simulink model "Altitudecontrolnewscheme"  (R2016a)
settings: Solver=VariableStepAuto  StartTime=0.0  StopTime=10  FixedStep=Ts  RelTol=1e-3
model workspace (MAT data in the model file):
  AC_ATTITUDE_ACCEL_Y_CONTROLLER_MAX_RADSS = Simulink.Signal
  AC_ATTITUDE_ACCEL_Y_CONTROLLER_MAX_RADSS.DataType = 'double'
  AC_ATTITUDE_ACCEL_Y_CONTROLLER_MAX_RADSS.Dimensions = 1
  AC_ATTITUDE_ACCEL_Y_CONTROLLER_MAX_RADSS.DimensionsMode = 'auto'
  AC_ATTITUDE_ACCEL_Y_CONTROLLER_MAX_RADSS.Complexity = 'real'
  AC_ATTITUDE_ACCEL_Y_CONTROLLER_MAX_RADSS.SampleTime = -1
  AC_ATTITUDE_ACCEL_Y_CONTROLLER_MAX_RADSS.SamplingMode = 'Sample based'
  AC_ATTITUDE_ACCEL_Y_CONTROLLER_MAX_RADSS.InitialValue = '0.5'
  AC_ATTITUDE_CONTROL_MAX = Simulink.Signal
  AC_ATTITUDE_CONTROL_MAX.DataType = 'double'
  AC_ATTITUDE_CONTROL_MAX.Dimensions = 1
  AC_ATTITUDE_CONTROL_MAX.DimensionsMode = 'auto'
  AC_ATTITUDE_CONTROL_MAX.Complexity = 'real'
  AC_ATTITUDE_CONTROL_MAX.SampleTime = -1
  AC_ATTITUDE_CONTROL_MAX.SamplingMode = 'Sample based'
  AC_ATTITUDE_CONTROL_MAX.InitialValue = '0.5'
  AC_ATTITUDE_THRUST_ERROR_ANGLE = Simulink.Signal
  AC_ATTITUDE_THRUST_ERROR_ANGLE.DataType = 'double'
  AC_ATTITUDE_THRUST_ERROR_ANGLE.Dimensions = 1
  AC_ATTITUDE_THRUST_ERROR_ANGLE.DimensionsMode = 'auto'
  AC_ATTITUDE_THRUST_ERROR_ANGLE.Complexity = 'real'
  AC_ATTITUDE_THRUST_ERROR_ANGLE.SampleTime = -1
  AC_ATTITUDE_THRUST_ERROR_ANGLE.SamplingMode = 'Sample based'
  AC_ATTITUDE_THRUST_ERROR_ANGLE.InitialValue = '1000'
  ROLL_PITCH_INPUT_MAX = Simulink.Signal
  ROLL_PITCH_INPUT_MAX.DataType = 'double'
  ROLL_PITCH_INPUT_MAX.Dimensions = 1
  ROLL_PITCH_INPUT_MAX.DimensionsMode = 'auto'
  ROLL_PITCH_INPUT_MAX.Complexity = 'real'
  ROLL_PITCH_INPUT_MAX.SampleTime = -1
  ROLL_PITCH_INPUT_MAX.SamplingMode = 'Sample based'
  ROLL_PITCH_INPUT_MAX.InitialValue = '3000'
  Sig = Simulink.Signal
  Sig.DataType = 'auto'
  Sig.Dimensions = -1
  Sig.DimensionsMode = 'auto'
  Sig.Complexity = 'auto'
  Sig.SampleTime = -1
  Sig.SamplingMode = 'auto'
  Sig1 = Simulink.Signal
  Sig1.DataType = 'auto'
  Sig1.Dimensions = -1
  Sig1.DimensionsMode = 'auto'
  Sig1.Complexity = 'auto'
  Sig1.SampleTime = -1
  Sig1.SamplingMode = 'auto'
  acro_yaw_p = Simulink.Signal
  acro_yaw_p.DataType = 'double'
  acro_yaw_p.Dimensions = 1
  acro_yaw_p.DimensionsMode = 'auto'
  acro_yaw_p.Complexity = 'real'
  acro_yaw_p.SampleTime = -1
  acro_yaw_p.SamplingMode = 'Sample based'
  acro_yaw_p.InitialValue = '45'
  angle_max = Simulink.Signal
  angle_max.DataType = 'double'
  angle_max.Dimensions = 1
  angle_max.DimensionsMode = 'auto'
  angle_max.Complexity = 'real'
  angle_max.SampleTime = -1
  angle_max.SamplingMode = 'Sample based'
  angle_max.InitialValue = '3000'
  attitude_target_ang_vel = Simulink.Signal
  attitude_target_ang_vel.DataType = 'double'
  attitude_target_ang_vel.Dimensions = 3
  attitude_target_ang_vel.DimensionsMode = 'auto'
  attitude_target_ang_vel.Complexity = 'real'
  attitude_target_ang_vel.SampleTime = -1
  attitude_target_ang_vel.SamplingMode = 'Sample based'
  attitude_target_ang_vel.InitialValue = '[0 0 0]'
  attitude_target_euler_angle_x = Simulink.Signal
  attitude_target_euler_angle_x.DataType = 'double'
  attitude_target_euler_angle_x.Dimensions = 1
  attitude_target_euler_angle_x.DimensionsMode = 'auto'
  attitude_target_euler_angle_x.Complexity = 'real'
  attitude_target_euler_angle_x.SampleTime = -1
  attitude_target_euler_angle_x.SamplingMode = 'Sample based'
  attitude_target_euler_angle_x.InitialValue = '0'
  attitude_target_euler_angle_y = Simulink.Signal
  attitude_target_euler_angle_y.DataType = 'double'
  attitude_target_euler_angle_y.Dimensions = 1
  attitude_target_euler_angle_y.DimensionsMode = 'auto'
  attitude_target_euler_angle_y.Complexity = 'real'
  attitude_target_euler_angle_y.SampleTime = -1
  attitude_target_euler_angle_y.SamplingMode = 'Sample based'
  attitude_target_euler_angle_y.InitialValue = '0'
  attitude_target_euler_angle_z = Simulink.Signal
  attitude_target_euler_angle_z.DataType = 'double'
  attitude_target_euler_angle_z.Dimensions = 1
  attitude_target_euler_angle_z.DimensionsMode = 'auto'
  attitude_target_euler_angle_z.Complexity = 'real'
  attitude_target_euler_angle_z.SampleTime = -1
  attitude_target_euler_angle_z.SamplingMode = 'Sample based'
  attitude_target_euler_angle_z.InitialValue = '0'
  attitude_target_euler_rate = Simulink.Signal
  attitude_target_euler_rate.DataType = 'double'
  attitude_target_euler_rate.Dimensions = 3
  attitude_target_euler_rate.DimensionsMode = 'auto'
  attitude_target_euler_rate.Complexity = 'real'
  attitude_target_euler_rate.SampleTime = -1
  attitude_target_euler_rate.SamplingMode = 'Sample based'
  attitude_target_euler_rate.InitialValue = '[0 0 0]'
  attitude_target_quat = Simulink.Signal
  attitude_target_quat.DataType = 'double'
  attitude_target_quat.Dimensions = 4
  attitude_target_quat.DimensionsMode = 'auto'
  attitude_target_quat.Complexity = 'real'
  attitude_target_quat.SampleTime = -1
  attitude_target_quat.SamplingMode = 'Sample based'
  attitude_target_quat.InitialValue = '[1 0 0 0]'
  attitude_vehicle_quat = Simulink.Signal
  attitude_vehicle_quat.DataType = 'double'
  attitude_vehicle_quat.Dimensions = 4
  attitude_vehicle_quat.DimensionsMode = 'auto'
  attitude_vehicle_quat.Complexity = 'real'
  attitude_vehicle_quat.SampleTime = -1
  attitude_vehicle_quat.SamplingMode = 'Sample based'
  attitude_vehicle_quat.InitialValue = '[1 0 0 0]'
  dt = Simulink.Signal
  dt.DataType = 'double'
  dt.Dimensions = 1
  dt.DimensionsMode = 'auto'
  dt.Complexity = 'real'
  dt.SampleTime = -1
  dt.SamplingMode = 'Sample based'
  dt.InitialValue = '0.01'
  false = 0
  limit_roll_pitch = Simulink.Signal
  limit_roll_pitch.DataType = 'double'
  limit_roll_pitch.Dimensions = 1
  limit_roll_pitch.DimensionsMode = 'auto'
  limit_roll_pitch.Complexity = 'real'
  limit_roll_pitch.SampleTime = -1
  limit_roll_pitch.SamplingMode = 'Sample based'
  limit_roll_pitch.InitialValue = '0.0'
  limit_throttle_upper = Simulink.Signal
  limit_throttle_upper.DataType = 'logical'
  limit_throttle_upper.Dimensions = 1
  limit_throttle_upper.DimensionsMode = 'auto'
  limit_throttle_upper.Complexity = 'real'
  limit_throttle_upper.SampleTime = -1
  limit_throttle_upper.SamplingMode = 'Sample based'
  limit_throttle_upper.InitialValue = '0'
  limit_yaw = Simulink.Signal
  limit_yaw.DataType = 'double'
  limit_yaw.Dimensions = 1
  limit_yaw.DimensionsMode = 'auto'
  limit_yaw.Complexity = 'real'
  limit_yaw.SampleTime = -1
  limit_yaw.SamplingMode = 'Sample based'
  limit_yaw.InitialValue = '0'
  loop_rate = Simulink.Signal
  loop_rate.DataType = 'double'
  loop_rate.Dimensions = 1
  loop_rate.DimensionsMode = 'auto'
  loop_rate.Complexity = 'real'
  loop_rate.SampleTime = -1
  loop_rate.SamplingMode = 'Sample based'
  loop_rate.InitialValue = '100'
  pitch_attitude_kP = Simulink.Signal
  pitch_attitude_kP.DataType = 'double'
  pitch_attitude_kP.Dimensions = 1
  pitch_attitude_kP.DimensionsMode = 'auto'
  pitch_attitude_kP.Complexity = 'real'
  pitch_attitude_kP.SampleTime = -1
  pitch_attitude_kP.SamplingMode = 'Sample based'
  pitch_attitude_kP.InitialValue = '20'
  pitch_factor = Simulink.Signal
  pitch_factor.DataType = 'double'
  pitch_factor.Dimensions = 4
  pitch_factor.DimensionsMode = 'auto'
  pitch_factor.Complexity = 'real'
  pitch_factor.SampleTime = -1
  pitch_factor.SamplingMode = 'Sample based'
  pitch_factor.InitialValue = '[cos(deg2rad(15)) -cos(deg2rad(15)) cos(deg2rad(15)) -cos(deg2rad(15))]'
  pitch_rate_derivative = Simulink.Signal
  pitch_rate_derivative.DataType = 'double'
  pitch_rate_derivative.Dimensions = 1
  pitch_rate_derivative.DimensionsMode = 'auto'
  pitch_rate_derivative.Complexity = 'real'
  pitch_rate_derivative.SampleTime = -1
  pitch_rate_derivative.SamplingMode = 'Sample based'
  pitch_rate_derivative.InitialValue = '0'
  pitch_rate_error_rads = Simulink.Signal
  pitch_rate_error_rads.DataType = 'double'
  pitch_rate_error_rads.Dimensions = 1
  pitch_rate_error_rads.DimensionsMode = 'auto'
  pitch_rate_error_rads.Complexity = 'real'
  pitch_rate_error_rads.SampleTime = -1
  pitch_rate_error_rads.SamplingMode = 'Sample based'
  pitch_rate_error_rads.InitialValue = '0'
  pitch_rate_filt_hz = Simulink.Signal
  pitch_rate_filt_hz.DataType = 'double'
  pitch_rate_filt_hz.Dimensions = 1
  pitch_rate_filt_hz.DimensionsMode = 'auto'
  pitch_rate_filt_hz.Complexity = 'real'
  pitch_rate_filt_hz.SampleTime = -1
  pitch_rate_filt_hz.SamplingMode = 'Sample based'
  pitch_rate_filt_hz.InitialValue = '1/(2*pi)'
  pitch_rate_imax = Simulink.Signal
  pitch_rate_imax.DataType = 'double'
  pitch_rate_imax.Dimensions = 1
  pitch_rate_imax.DimensionsMode = 'auto'
  pitch_rate_imax.Complexity = 'real'
  pitch_rate_imax.SampleTime = -1
  pitch_rate_imax.SamplingMode = 'Sample based'
  pitch_rate_imax.InitialValue = '200'
  pitch_rate_integrator = Simulink.Signal
  pitch_rate_integrator.DataType = 'double'
  pitch_rate_integrator.Dimensions = 1
  pitch_rate_integrator.DimensionsMode = 'auto'
  pitch_rate_integrator.Complexity = 'real'
  pitch_rate_integrator.SampleTime = -1
  pitch_rate_integrator.SamplingMode = 'Sample based'
  pitch_rate_integrator.InitialValue = '0'
  pitch_rate_kD = Simulink.Signal
  pitch_rate_kD.DataType = 'double'
  pitch_rate_kD.Dimensions = 1
  pitch_rate_kD.DimensionsMode = 'auto'
  pitch_rate_kD.Complexity = 'real'
  pitch_rate_kD.SampleTime = -1
  pitch_rate_kD.SamplingMode = 'Sample based'
  pitch_rate_kD.InitialValue = '0.004'
  pitch_rate_kI = Simulink.Signal
  pitch_rate_kI.DataType = 'double'
  pitch_rate_kI.Dimensions = 1
  pitch_rate_kI.DimensionsMode = 'auto'
  pitch_rate_kI.Complexity = 'real'
  pitch_rate_kI.SampleTime = -1
  pitch_rate_kI.SamplingMode = 'Sample based'
  pitch_rate_kI.InitialValue = '0.1'
  pitch_rate_kP = Simulink.Signal
  pitch_rate_kP.DataType = 'double'
  pitch_rate_kP.Dimensions = 1
  pitch_rate_kP.DimensionsMode = 'auto'
  pitch_rate_kP.Complexity = 'real'
  pitch_rate_kP.SampleTime = -1
  pitch_rate_kP.SamplingMode = 'Sample based'
  pitch_rate_kP.InitialValue = '0.5'
  pitch_rate_last_input = Simulink.Signal
  pitch_rate_last_input.DataType = 'double'
  pitch_rate_last_input.Dimensions = 1
  pitch_rate_last_input.DimensionsMode = 'auto'
  pitch_rate_last_input.Complexity = 'real'
  pitch_rate_last_input.SampleTime = -1
  pitch_rate_last_input.SamplingMode = 'Sample based'
  pitch_rate_last_input.InitialValue = '0'
  pitch_rate_proportional = Simulink.Signal
  pitch_rate_proportional.DataType = 'double'
  pitch_rate_proportional.Dimensions = 1
  pitch_rate_proportional.DimensionsMode = 'auto'
  pitch_rate_proportional.Complexity = 'real'
  pitch_rate_proportional.SampleTime = -1
  pitch_rate_proportional.SamplingMode = 'Sample based'
  pitch_rate_proportional.InitialValue = '0'
  pwm_max = Simulink.Signal
  pwm_max.DataType = 'double'
  pwm_max.Dimensions = 1
  pwm_max.DimensionsMode = 'auto'
  pwm_max.Complexity = 'real'
  pwm_max.SampleTime = -1
  pwm_max.SamplingMode = 'Sample based'
  pwm_max.InitialValue = '2000'
  pwm_min = Simulink.Signal
  pwm_min.DataType = 'double'
  pwm_min.Dimensions = 1
  pwm_min.DimensionsMode = 'auto'
  pwm_min.Complexity = 'real'
  pwm_min.SampleTime = -1
  pwm_min.SamplingMode = 'Sample based'
  pwm_min.InitialValue = '1039'
  rate_bf_ff_enabled = Simulink.Signal
  rate_bf_ff_enabled.DataType = 'double'
  rate_bf_ff_enabled.Dimensions = 1
  rate_bf_ff_enabled.DimensionsMode = 'auto'
  rate_bf_ff_enabled.Complexity = 'real'
  rate_bf_ff_enabled.SampleTime = -1
  rate_bf_ff_enabled.SamplingMode = 'Sample based'
  rate_bf_ff_enabled.InitialValue = '0'
  rate_target_ang_vel = Simulink.Signal
  rate_target_ang_vel.DataType = 'double'
  rate_target_ang_vel.Dimensions = 3
  rate_target_ang_vel.DimensionsMode = 'auto'
  rate_target_ang_vel.Complexity = 'real'
  rate_target_ang_vel.SampleTime = -1
  rate_target_ang_vel.SamplingMode = 'Sample based'
  rate_target_ang_vel.InitialValue = '[0 0 0]'
  roll_attitude_kP = Simulink.Signal
  roll_attitude_kP.DataType = 'double'
  roll_attitude_kP.Dimensions = 1
  roll_attitude_kP.DimensionsMode = 'auto'
  roll_attitude_kP.Complexity = 'real'
  roll_attitude_kP.SampleTime = -1
  roll_attitude_kP.SamplingMode = 'Sample based'
  roll_attitude_kP.InitialValue = '20'
  roll_factor = Simulink.Signal
  roll_factor.DataType = 'double'
  roll_factor.Dimensions = 4
  roll_factor.DimensionsMode = 'auto'
  roll_factor.Complexity = 'real'
  roll_factor.SampleTime = -1
  roll_factor.SamplingMode = 'Sample based'
  roll_factor.InitialValue = '[-sin(deg2rad(15)) sin(deg2rad(15)) sin(deg2rad(15)) -sin(deg2rad(15))]'
  roll_rate_derivative = Simulink.Signal
  roll_rate_derivative.DataType = 'double'
  roll_rate_derivative.Dimensions = 1
  roll_rate_derivative.DimensionsMode = 'auto'
  roll_rate_derivative.Complexity = 'real'
  roll_rate_derivative.SampleTime = -1
  roll_rate_derivative.SamplingMode = 'Sample based'
  roll_rate_derivative.InitialValue = '0'
  roll_rate_error_rads = Simulink.Signal
  roll_rate_error_rads.DataType = 'double'
  roll_rate_error_rads.Dimensions = 1
  roll_rate_error_rads.DimensionsMode = 'auto'
  roll_rate_error_rads.Complexity = 'real'
  roll_rate_error_rads.SampleTime = -1
  roll_rate_error_rads.SamplingMode = 'Sample based'
  roll_rate_error_rads.InitialValue = '0'
  roll_rate_filt_hz = Simulink.Signal
  roll_rate_filt_hz.DataType = 'double'
  roll_rate_filt_hz.Dimensions = 1
  roll_rate_filt_hz.DimensionsMode = 'auto'
  roll_rate_filt_hz.Complexity = 'real'
  roll_rate_filt_hz.SampleTime = -1
  roll_rate_filt_hz.SamplingMode = 'Sample based'
  roll_rate_filt_hz.InitialValue = '1/(2*pi)'
  roll_rate_imax = Simulink.Signal
  roll_rate_imax.DataType = 'double'
  roll_rate_imax.Dimensions = 1
  roll_rate_imax.DimensionsMode = 'auto'
  roll_rate_imax.Complexity = 'real'
  roll_rate_imax.SampleTime = -1
  roll_rate_imax.SamplingMode = 'Sample based'
  roll_rate_imax.InitialValue = '200'
  roll_rate_integrator = Simulink.Signal
  roll_rate_integrator.DataType = 'double'
  roll_rate_integrator.Dimensions = 1
  roll_rate_integrator.DimensionsMode = 'auto'
  roll_rate_integrator.Complexity = 'real'
  roll_rate_integrator.SampleTime = -1
  roll_rate_integrator.SamplingMode = 'Sample based'
  roll_rate_integrator.InitialValue = '0'
  roll_rate_kD = Simulink.Signal
  roll_rate_kD.DataType = 'double'
  roll_rate_kD.Dimensions = 1
  roll_rate_kD.DimensionsMode = 'auto'
  roll_rate_kD.Complexity = 'real'
  roll_rate_kD.SampleTime = -1
  roll_rate_kD.SamplingMode = 'Sample based'
  roll_rate_kD.InitialValue = '0.004'
  roll_rate_kI = Simulink.Signal
  roll_rate_kI.DataType = 'double'
  roll_rate_kI.Dimensions = 1
  roll_rate_kI.DimensionsMode = 'auto'
  roll_rate_kI.Complexity = 'real'
  roll_rate_kI.SampleTime = -1
  roll_rate_kI.SamplingMode = 'Sample based'
  roll_rate_kI.InitialValue = '0.1'
  roll_rate_kP = Simulink.Signal
  roll_rate_kP.DataType = 'double'
  roll_rate_kP.Dimensions = 1
  roll_rate_kP.DimensionsMode = 'auto'
  roll_rate_kP.Complexity = 'real'
  roll_rate_kP.SampleTime = -1
  roll_rate_kP.SamplingMode = 'Sample based'
  roll_rate_kP.InitialValue = '1'
  roll_rate_last_input = Simulink.Signal
  roll_rate_last_input.DataType = 'double'
  roll_rate_last_input.Dimensions = 1
  roll_rate_last_input.DimensionsMode = 'auto'
  roll_rate_last_input.Complexity = 'real'
  roll_rate_last_input.SampleTime = -1
  roll_rate_last_input.SamplingMode = 'Sample based'
  roll_rate_last_input.InitialValue = '0'
  roll_rate_proportional = Simulink.Signal
  roll_rate_proportional.DataType = 'double'
  roll_rate_proportional.Dimensions = 1
  roll_rate_proportional.DimensionsMode = 'auto'
  roll_rate_proportional.Complexity = 'real'
  roll_rate_proportional.SampleTime = -1
  roll_rate_proportional.SamplingMode = 'Sample based'
  roll_rate_proportional.InitialValue = '0'
  spin_max = Simulink.Signal
  spin_max.DataType = 'double'
  spin_max.Dimensions = 1
  spin_max.DimensionsMode = 'auto'
  spin_max.Complexity = 'real'
  spin_max.SampleTime = -1
  spin_max.SamplingMode = 'Sample based'
  spin_max.InitialValue = '0.95'
  spin_min = Simulink.Signal
  spin_min.DataType = 'double'
  spin_min.Dimensions = 1
  spin_min.DimensionsMode = 'auto'
  spin_min.Complexity = 'real'
  spin_min.SampleTime = -1
  spin_min.SamplingMode = 'Sample based'
  spin_min.InitialValue = '0.15'
  throttle_avg_max = Simulink.Signal
  throttle_avg_max.DataType = 'double'
  throttle_avg_max.Dimensions = 1
  throttle_avg_max.DimensionsMode = 'auto'
  throttle_avg_max.Complexity = 'real'
  throttle_avg_max.SampleTime = -1
  throttle_avg_max.SamplingMode = 'Sample based'
  throttle_avg_max.InitialValue = '0'
  throttle_filter_cutoff_freq = Simulink.Signal
  throttle_filter_cutoff_freq.DataType = 'double'
  throttle_filter_cutoff_freq.Dimensions = 1
  throttle_filter_cutoff_freq.DimensionsMode = 'auto'
  throttle_filter_cutoff_freq.Complexity = 'real'
  throttle_filter_cutoff_freq.SampleTime = -1
  throttle_filter_cutoff_freq.SamplingMode = 'Sample based'
  throttle_filter_cutoff_freq.InitialValue = '0.5'
  throttle_filter_output = Simulink.Signal
  throttle_filter_output.DataType = 'double'
  throttle_filter_output.Dimensions = 1
  throttle_filter_output.DimensionsMode = 'auto'
  throttle_filter_output.Complexity = 'real'
  throttle_filter_output.SampleTime = -1
  throttle_filter_output.SamplingMode = 'Sample based'
  throttle_filter_output.InitialValue = '0'
  throttle_in = Simulink.Signal
  throttle_in.DataType = 'double'
  throttle_in.Dimensions = 1
  throttle_in.DimensionsMode = 'auto'
  throttle_in.Complexity = 'real'
  throttle_in.SampleTime = -1
  throttle_in.SamplingMode = 'Sample based'
  throttle_in.InitialValue = '0'
  throttle_rpy_mix = Simulink.Signal
  throttle_rpy_mix.DataType = 'double'
  throttle_rpy_mix.Dimensions = 1
  throttle_rpy_mix.DimensionsMode = 'auto'
  throttle_rpy_mix.Complexity = 'real'
  throttle_rpy_mix.SampleTime = -1
  throttle_rpy_mix.SamplingMode = 'Sample based'
  throttle_rpy_mix.InitialValue = '0'
  throttle_rpy_mix_desired = Simulink.Signal
  throttle_rpy_mix_desired.DataType = 'double'
  throttle_rpy_mix_desired.Dimensions = 1
  throttle_rpy_mix_desired.DimensionsMode = 'auto'
  throttle_rpy_mix_desired.Complexity = 'real'
  throttle_rpy_mix_desired.SampleTime = -1
  throttle_rpy_mix_desired.SamplingMode = 'Sample based'
  throttle_rpy_mix_desired.InitialValue = '0'
  throttle_thrust = Simulink.Signal
  throttle_thrust.DataType = 'double'
  throttle_thrust.Dimensions = 1
  throttle_thrust.DimensionsMode = 'auto'
  throttle_thrust.Complexity = 'real'
  throttle_thrust.SampleTime = -1
  throttle_thrust.SamplingMode = 'Sample based'
  throttle_thrust.InitialValue = '0'
  throttle_thrust_best_rpy = Simulink.Signal
  throttle_thrust_best_rpy.DataType = 'double'
  throttle_thrust_best_rpy.Dimensions = 1
  throttle_thrust_best_rpy.DimensionsMode = 'auto'
  throttle_thrust_best_rpy.Complexity = 'real'
  throttle_thrust_best_rpy.SampleTime = -1
  throttle_thrust_best_rpy.SamplingMode = 'Sample based'
  throttle_thrust_best_rpy.InitialValue = '0'
  throttle_thrust_max = Simulink.Signal
  throttle_thrust_max.DataType = 'double'
  throttle_thrust_max.Dimensions = 1
  throttle_thrust_max.DimensionsMode = 'auto'
  throttle_thrust_max.Complexity = 'real'
  throttle_thrust_max.SampleTime = -1
  throttle_thrust_max.SamplingMode = 'Sample based'
  throttle_thrust_max.InitialValue = '1'
  thrust_error_angle = Simulink.Signal
  thrust_error_angle.DataType = 'double'
  thrust_error_angle.Dimensions = 1
  thrust_error_angle.DimensionsMode = 'auto'
  thrust_error_angle.Complexity = 'real'
  thrust_error_angle.SampleTime = -1
  thrust_error_angle.SamplingMode = 'Sample based'
  thrust_error_angle.InitialValue = '0'
  thrust_rpyt_out = Simulink.Signal
  thrust_rpyt_out.DataType = 'double'
  thrust_rpyt_out.Dimensions = 4
  thrust_rpyt_out.DimensionsMode = 'auto'
  thrust_rpyt_out.Complexity = 'real'
  thrust_rpyt_out.SampleTime = -1
  thrust_rpyt_out.SamplingMode = 'Sample based'
  thrust_rpyt_out.InitialValue = '[0 0 0 0]'
  true = 1
  use_ff_and_input_shaping = Simulink.Signal
  use_ff_and_input_shaping.DataType = 'double'
  use_ff_and_input_shaping.Dimensions = 1
  use_ff_and_input_shaping.DimensionsMode = 'auto'
  use_ff_and_input_shaping.Complexity = 'real'
  use_ff_and_input_shaping.SampleTime = -1
  use_ff_and_input_shaping.SamplingMode = 'Sample based'
  use_ff_and_input_shaping.InitialValue = '0'
  variableType = 'S'
  yaw_allowed = Simulink.Signal
  yaw_allowed.DataType = 'double'
  yaw_allowed.Dimensions = 1
  yaw_allowed.DimensionsMode = 'auto'
  yaw_allowed.Complexity = 'real'
  yaw_allowed.SampleTime = -1
  yaw_allowed.SamplingMode = 'Sample based'
  yaw_allowed.InitialValue = '1'
  yaw_attitude_kP = Simulink.Signal
  yaw_attitude_kP.DataType = 'double'
  yaw_attitude_kP.Dimensions = 1
  yaw_attitude_kP.DimensionsMode = 'auto'
  yaw_attitude_kP.Complexity = 'real'
  yaw_attitude_kP.SampleTime = -1
  yaw_attitude_kP.SamplingMode = 'Sample based'
  yaw_attitude_kP.InitialValue = '4.5'
  yaw_factor = Simulink.Signal
  yaw_factor.DataType = 'double'
  yaw_factor.Dimensions = 4
  yaw_factor.DimensionsMode = 'auto'
  yaw_factor.Complexity = 'real'
  yaw_factor.SampleTime = -1
  yaw_factor.SamplingMode = 'Sample based'
  yaw_factor.InitialValue = '[0.1 0.1 -0.1 -0.1]'
  yaw_headroom = Simulink.Signal
  yaw_headroom.DataType = 'double'
  yaw_headroom.Dimensions = 1
  yaw_headroom.DimensionsMode = 'auto'
  yaw_headroom.Complexity = 'real'
  yaw_headroom.SampleTime = -1
  yaw_headroom.SamplingMode = 'Sample based'
  yaw_headroom.InitialValue = '200'
  yaw_rate_derivative = Simulink.Signal
  yaw_rate_derivative.DataType = 'double'
  yaw_rate_derivative.Dimensions = 1
  yaw_rate_derivative.DimensionsMode = 'auto'
  yaw_rate_derivative.Complexity = 'real'
  yaw_rate_derivative.SampleTime = -1
  yaw_rate_derivative.SamplingMode = 'Sample based'
  yaw_rate_derivative.InitialValue = '0'
  yaw_rate_error_rads = Simulink.Signal
  yaw_rate_error_rads.DataType = 'double'
  yaw_rate_error_rads.Dimensions = 1
  yaw_rate_error_rads.DimensionsMode = 'auto'
  yaw_rate_error_rads.Complexity = 'real'
  yaw_rate_error_rads.SampleTime = -1
  yaw_rate_error_rads.SamplingMode = 'Sample based'
  yaw_rate_error_rads.InitialValue = '0'
  yaw_rate_filt_hz = Simulink.Signal
  yaw_rate_filt_hz.DataType = 'double'
  yaw_rate_filt_hz.Dimensions = 1
  yaw_rate_filt_hz.DimensionsMode = 'auto'
  yaw_rate_filt_hz.Complexity = 'real'
  yaw_rate_filt_hz.SampleTime = -1
  yaw_rate_filt_hz.SamplingMode = 'Sample based'
  yaw_rate_filt_hz.InitialValue = '1/(2*pi)'
  yaw_rate_imax = Simulink.Signal
  yaw_rate_imax.DataType = 'double'
  yaw_rate_imax.Dimensions = 1
  yaw_rate_imax.DimensionsMode = 'auto'
  yaw_rate_imax.Complexity = 'real'
  yaw_rate_imax.SampleTime = -1
  yaw_rate_imax.SamplingMode = 'Sample based'
  yaw_rate_imax.InitialValue = '200'
  yaw_rate_integrator = Simulink.Signal
  yaw_rate_integrator.DataType = 'double'
  yaw_rate_integrator.Dimensions = 1
  yaw_rate_integrator.DimensionsMode = 'auto'
  yaw_rate_integrator.Complexity = 'real'
  yaw_rate_integrator.SampleTime = -1
  yaw_rate_integrator.SamplingMode = 'Sample based'
  yaw_rate_integrator.InitialValue = '0'
  yaw_rate_kD = Simulink.Signal
  yaw_rate_kD.DataType = 'double'
  yaw_rate_kD.Dimensions = 1
  yaw_rate_kD.DimensionsMode = 'auto'
  yaw_rate_kD.Complexity = 'real'
  yaw_rate_kD.SampleTime = -1
  yaw_rate_kD.SamplingMode = 'Sample based'
  yaw_rate_kD.InitialValue = '5'
  yaw_rate_kI = Simulink.Signal
  yaw_rate_kI.DataType = 'double'
  yaw_rate_kI.Dimensions = 1
  yaw_rate_kI.DimensionsMode = 'auto'
  yaw_rate_kI.Complexity = 'real'
  yaw_rate_kI.SampleTime = -1
  yaw_rate_kI.SamplingMode = 'Sample based'
  yaw_rate_kI.InitialValue = '0.1'
  yaw_rate_kP = Simulink.Signal
  yaw_rate_kP.DataType = 'double'
  yaw_rate_kP.Dimensions = 1
  yaw_rate_kP.DimensionsMode = 'auto'
  yaw_rate_kP.Complexity = 'real'
  yaw_rate_kP.SampleTime = -1
  yaw_rate_kP.SamplingMode = 'Sample based'
  yaw_rate_kP.InitialValue = '0.2'
  yaw_rate_last_input = Simulink.Signal
  yaw_rate_last_input.DataType = 'double'
  yaw_rate_last_input.Dimensions = 1
  yaw_rate_last_input.DimensionsMode = 'auto'
  yaw_rate_last_input.Complexity = 'real'
  yaw_rate_last_input.SampleTime = -1
  yaw_rate_last_input.SamplingMode = 'Sample based'
  yaw_rate_last_input.InitialValue = '0'
  yaw_rate_proportional = Simulink.Signal
  yaw_rate_proportional.DataType = 'double'
  yaw_rate_proportional.Dimensions = 1
  yaw_rate_proportional.DimensionsMode = 'auto'
  yaw_rate_proportional.Complexity = 'real'
  yaw_rate_proportional.SampleTime = -1
  yaw_rate_proportional.SamplingMode = 'Sample based'
  yaw_rate_proportional.InitialValue = '0'
undefined symbols (not defined in the file or in its folder): dtzoh, Ts
libraries: aerolib6dof2 x1, simulink x1, aerolibconvert2 x1
settings Model: Creator=s121814  LastModifiedBy=GusBus
settings SolverCC: ZeroCrossControl=DisableAll
settings DataIOCC: SaveFormat=Array  SaveState=on

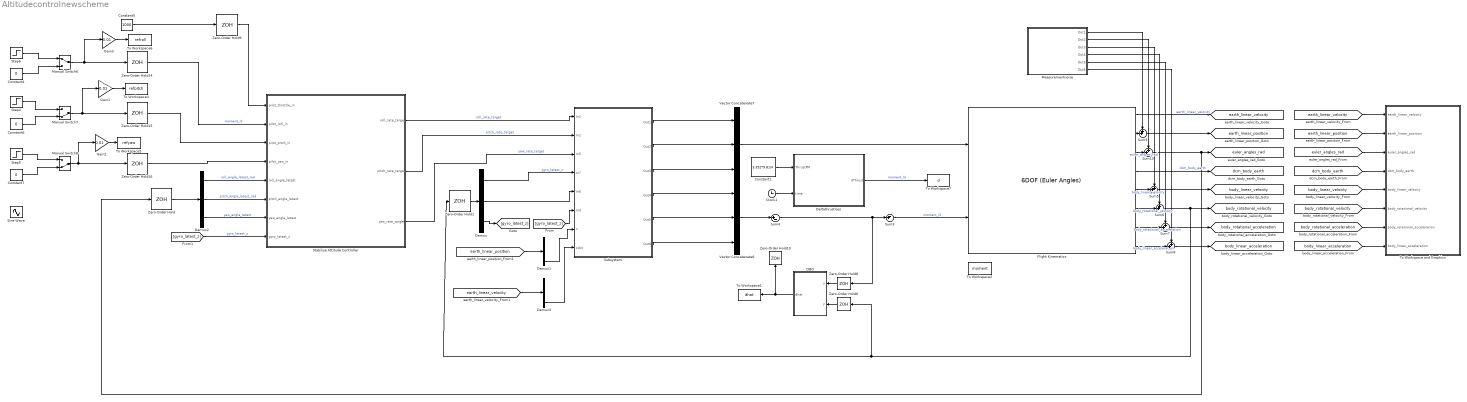
== system Altitudecontrolnewscheme ==
  Clock1 : Clock
  Constant1 : Constant  Value=3.352*9.81/4  SampleTime=Ts
  Constant4 : Constant  Value=0  SampleTime=0
  Constant5 : Constant  Value=1000  SampleTime=Ts
  Constant6 : Constant  Value=0  SampleTime=0
  Constant7 : Constant  Value=0  SampleTime=0
  DBO : Subsystem
  Deltathrustloss : MATLAB Function  TreatAsAtomicUnit=on
  Demux{,1..3} (4 alike) : Demux  Outputs=3
  Flight Kinematics : aerolib6dof2/6DOF (Euler Angles)  units=Metric (MKS)  mtype=Fixed  rep=Euler Angles  xme_0=[0 0 0]  Vm_0=[0 0 0]  eul_0=[0 0 0]  pm_0=[0 0 0]  mass_0=3.352  mass_e=0.5  mass_f=2.0  inertia=[0.025028 0 0; 0 0.16926 0; 0 0 0.170197]  inertia_e=eye(3)  inertia_f=2*eye(3)  k_quat=1.0  vre_flag=on
  Gain1 : Gain  Gain=0.01
  Gain2 : Gain  Gain=0.01
  Gain3 : Gain  Gain=0.01
  Manual Switch6 : ManualSwitch
  Manual Switch7 : ManualSwitch  CurrentSetting=0
  Manual Switch8 : ManualSwitch  CurrentSetting=0
  "Measurementnoise " : Subsystem
  Sine Wave : Sin  Amplitude=100  SampleTime=0
  Stabilise Attitude Controller : MATLAB Function  TreatAsAtomicUnit=on
  Step4 : Step  Time=0.1  After=1000  SampleTime=0
  Step5 : Step  Time=0.1  After=1000  SampleTime=0
  Step6 : Step  Time=0.5  After=1000  SampleTime=0
  Subsystem : Subsystem
  Sum{5..10} (6 alike) : Sum  Inputs=++|
  Sum3 : Sum  Inputs=-+|
  Sum4 : Sum  Inputs=|+-
  To Workspace and Graphics : Subsystem
  To Workspace1 : ToWorkspace  VariableName=dhat  SampleTime=-1
  To Workspace2 : ToWorkspace  VariableName=moment  SampleTime=-1
  To Workspace4 : ToWorkspace  VariableName=refpitch  SampleTime=-1
  To Workspace5 : ToWorkspace  VariableName=refyaw  SampleTime=-1
  To Workspace6 : ToWorkspace  VariableName=refroll  SampleTime=-1
  To Workspace7 : ToWorkspace  VariableName=d  SampleTime=-1
  Vector Concatenate6 : Concatenate  NumInputs=3
  Vector Concatenate7 : Concatenate  NumInputs=3
  Zero-Order Hold{,1,6,8..10,14..16} (9 alike) : ZeroOrderHold  SampleTime=dtzoh
  tag scope: body_linear_acceleration=global, body_linear_velocity=global, body_rotational_acceleration=global, body_rotational_velocity=global, dcm_body_earth=global, earth_linear_position=global, earth_linear_velocity=global, euler_angles_rad=global
  wires:
  Constant5/1 -> Zero-Order Hold9/1
  [body_rotational_velocity] -> To Workspace and Graphics/6(body_rotational_velocity)
  [body_linear_acceleration] -> To Workspace and Graphics/8(body_linear_acceleration)
  [body_rotational_acceleration] -> To Workspace and Graphics/7(body_rotational_acceleration)
  [body_linear_velocity] -> To Workspace and Graphics/5(body_linear_velocity)
  [dcm_body_earth] -> To Workspace and Graphics/4(dcm_body_earth)
  [euler_angles_rad] -> To Workspace and Graphics/3(euler_angles_rad)
  [earth_linear_position] -> To Workspace and Graphics/2(earth_linear_position)
  [earth_linear_velocity] -> To Workspace and Graphics/1(earth_linear_velocity)
  Flight Kinematics/1 -> [earth_linear_velocity]  "earth_linear_velocity"
  Flight Kinematics/7 -> Sum7/2  "body_rotational_acceleration"
  Flight Kinematics/8 -> Sum8/2  "body_linear_acceleration"
  Demux2/1 -> Stabilise Attitude Controller/5(roll_angle_latest)  "roll_angle_latest_rad"
  Demux2/2 -> Stabilise Attitude Controller/6(pitch_angle_latest)  "pitch_angle_latest_rad"
  Demux2/3 -> Stabilise Attitude Controller/7(yaw_angle_latest)  "yaw_angle_latest"
  [gyro_latest_z] -> Stabilise Attitude Controller/8(gyro_latest_z)  "gyro_latest_z"
  Demux/3 -> [gyro_latest_z]
  Zero-Order Hold1/1 -> Demux/1
  Zero-Order Hold/1 -> Demux2/1
  Zero-Order Hold9/1 -> Stabilise Attitude Controller/1(pilot_throttle_in)
  Manual Switch7/1 -> Gain1/1, Zero-Order Hold15/1
  Zero-Order Hold16/1 -> Stabilise Attitude Controller/4(pilot_yaw_in)
  Zero-Order Hold15/1 -> Stabilise Attitude Controller/3(pilot_pitch_in)
  Vector Concatenate7/1 -> Flight Kinematics/1
  Flight Kinematics/4 -> [dcm_body_earth]  "dcm_body_earth"
  Flight Kinematics/5 -> Sum5/2  "body_linear_velocity"
  Constant6/1 -> Manual Switch7/2
  Step5/1 -> Manual Switch8/1
  Constant7/1 -> Manual Switch8/2
  Sum3/1 -> Flight Kinematics/2  "moment_l2"
  Sum4/1 -> Zero-Order Hold8/1, Sum3/2
  Vector Concatenate6/1 -> Sum4/1
  Sum10/1 -> Zero-Order Hold/1, [euler_angles_rad]
  Flight Kinematics/3 -> Sum10/2  "euler_angles_rad"
  Sum9/1 -> [earth_linear_position]
  Flight Kinematics/2 -> Sum9/2
  Sum5/1 -> [body_linear_velocity]
  Flight Kinematics/6 -> Sum6/2  "body_rotational_velocity"
  Sum6/1 -> Zero-Order Hold1/1, Zero-Order Hold6/1, [body_rotational_velocity]
  Sum7/1 -> [body_rotational_acceleration]
  Sum8/1 -> [body_linear_acceleration]
  DBO/1("dhat ") -> To Workspace1/1, Zero-Order Hold10/1
  Step6/1 -> Manual Switch6/1
  Zero-Order Hold14/1 -> Stabilise Attitude Controller/2(pilot_roll_in)  "moment_l2"
  Gain1/1 -> To Workspace4/1
  Constant4/1 -> Manual Switch6/2
  Zero-Order Hold6/1 -> DBO/2(y)
  Zero-Order Hold8/1 -> DBO/1("u ")
  Constant1/1 -> Deltathrustloss/1(ThrustPM)
  Stabilise Attitude Controller/1(roll_rate_target) -> Subsystem/1(In1)  "roll_rate_target"
  Stabilise Attitude Controller/2(pitch_rate_target) -> Subsystem/2(In2)  "pitch_rate_target"
  Subsystem/1(Out1) -> Vector Concatenate7/1
  Subsystem/2(Out2) -> Vector Concatenate7/2
  Subsystem/3(Out3) -> Vector Concatenate7/3
  Subsystem/4(Out4) -> Vector Concatenate6/1
  Subsystem/5(Out5) -> Vector Concatenate6/2
  Subsystem/6(Out6) -> Vector Concatenate6/3
  [gyro_latest_z] -> Subsystem/6(In3)
  Demux/2 -> Subsystem/5(In6)
  Demux/1 -> Subsystem/4(In7)  "gyro_latest_x"
  Stabilise Attitude Controller/3(yaw_rate_target) -> Subsystem/3(In5)  "yaw_rate_target"
  Clock1/1 -> Deltathrustloss/2(time)
  "Measurementnoise "/1(Out1) -> Sum9/1
  "Measurementnoise "/2(Out2) -> Sum10/1
  "Measurementnoise "/3(Out3) -> Sum5/1
  "Measurementnoise "/4(Out4) -> Sum6/1
  "Measurementnoise "/5(Out5) -> Sum7/1
  "Measurementnoise "/6(Out6) -> Sum8/1
  Step4/1 -> Manual Switch7/1
  Manual Switch8/1 -> Gain2/1, Zero-Order Hold16/1
  Gain2/1 -> To Workspace5/1
  Manual Switch6/1 -> Gain3/1, Zero-Order Hold14/1
  Gain3/1 -> To Workspace6/1
  Deltathrustloss/1(dThrust) -> To Workspace7/1  "moment_ld"
  [earth_linear_position] -> Demux1/1
  Demux1/3 -> Subsystem/7(z)
  [earth_linear_velocity] -> Demux3/1
  Demux3/3 -> Subsystem/8(zdot)

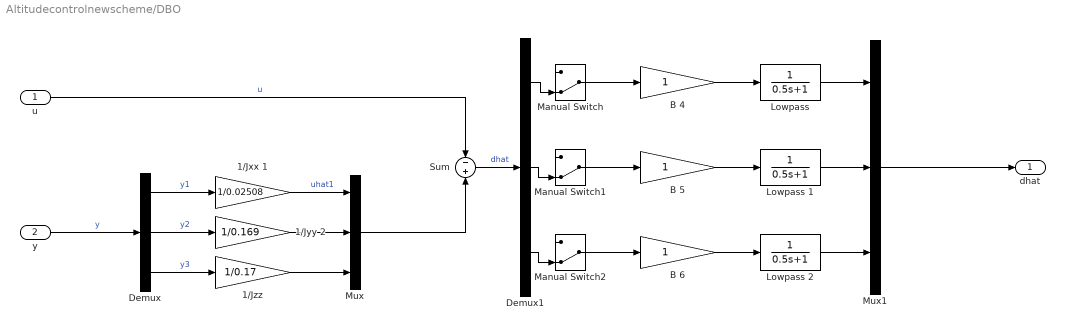
== system Altitudecontrolnewscheme/DBO ==
  "u " : Inport
  y : Inport  Port=2
  1/Jxx 1 : Gain  Gain=1/0.02508
  1/Jyy 2 : Gain  Gain=1/0.169
  1/Jzz : Gain  Gain=1/0.17
  B 4 : Gain
  B 5 : Gain
  B 6 : Gain
  Demux : Demux  Outputs=3
  Demux1 : Demux  Outputs=3
  "Lowpass " : TransferFcn  Denominator=[0.5 1]
  Lowpass 1 : TransferFcn  Denominator=[0.5 1]
  Lowpass 2 : TransferFcn  Denominator=[0.5 1]
  Manual Switch : ManualSwitch  CurrentSetting=0
  Manual Switch1 : ManualSwitch  CurrentSetting=0
  Manual Switch2 : ManualSwitch  CurrentSetting=0
  Mux : Mux  Inputs=3
  Mux1 : Mux  Inputs=3
  Sum : Sum  Inputs=-|+
  "dhat " : Outport
  wires:
  "u "/1 -> Sum/1  "u"
  y/1 -> Demux/1  "y"
  Demux/1 -> 1/Jxx 1/1  "y1"
  1/Jxx 1/1 -> Mux/1  "uhat1"
  Demux/2 -> 1/Jyy 2/1  "y2"
  1/Jyy 2/1 -> Mux/2
  Demux/3 -> 1/Jzz/1  "y3"
  1/Jzz/1 -> Mux/3
  Demux1/1 -> Manual Switch/2
  B 4/1 -> "Lowpass "/1
  Demux1/2 -> Manual Switch1/2
  B 5/1 -> Lowpass 1/1
  Demux1/3 -> Manual Switch2/2
  B 6/1 -> Lowpass 2/1
  Sum/1 -> Demux1/1  "dhat"
  Mux/1 -> Sum/2
  Mux1/1 -> "dhat "/1
  "Lowpass "/1 -> Mux1/1
  Manual Switch/1 -> B 4/1
  Lowpass 1/1 -> Mux1/2
  Lowpass 2/1 -> Mux1/3
  Manual Switch1/1 -> B 5/1
  Manual Switch2/1 -> B 6/1

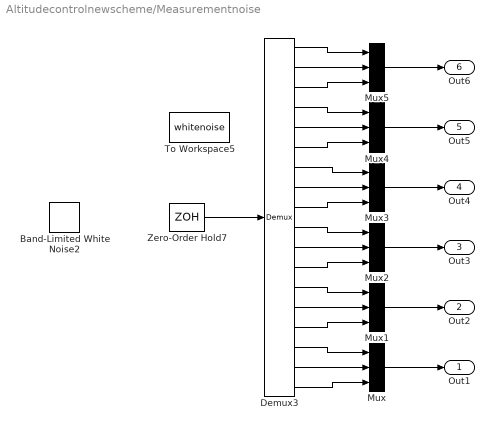
== system Altitudecontrolnewscheme/Measurementnoise  ==
  Band-Limited White Noise2 : simulink/Sources/Band-Limited White Noise  Cov=[0.00001 0.00001 0.00001 0.00001 0.00001 0.00001 0.00001 0.00001 0.00001 0.00001 0.00001 0.00001 0.00001 0.00001 0.00001 0.00001 0.00001 0.00001]*0.00001  Ts=Ts  seed=[23341 23341 23341 23341 23341 23341 23341 23341 23341 23341 23341 23341 23341 23341 23341 23341 23341 23341]
  Demux3 : Demux  Outputs=18
  Mux{,1..5} (6 alike) : Mux  Inputs=3
  To Workspace5 : ToWorkspace  VariableName=whitenoise  SampleTime=-1
  Zero-Order Hold7 : ZeroOrderHold  SampleTime=dtzoh
  Out1 : Outport
  Out2 : Outport  Port=2
  Out3 : Outport  Port=3
  Out4 : Outport  Port=4
  Out5 : Outport  Port=5
  Out6 : Outport  Port=6
  wires:
  Mux2/1 -> Out3/1
  Demux3/13 -> Mux1/1
  Demux3/1 -> Mux5/1
  Demux3/9 -> Mux3/3
  Demux3/7 -> Mux3/1
  Demux3/4 -> Mux4/1
  Demux3/18 -> Mux/3
  Demux3/5 -> Mux4/2
  Demux3/6 -> Mux4/3
  Demux3/11 -> Mux2/2
  Zero-Order Hold7/1 -> Demux3/1
  Mux/1 -> Out1/1
  Demux3/2 -> Mux5/2
  Demux3/12 -> Mux2/3
  Demux3/17 -> Mux/2
  Demux3/10 -> Mux2/1
  Demux3/3 -> Mux5/3
  Demux3/15 -> Mux1/3
  Mux1/1 -> Out2/1
  Demux3/8 -> Mux3/2
  Demux3/14 -> Mux1/2
  Demux3/16 -> Mux/1
  Mux4/1 -> Out5/1
  Mux5/1 -> Out6/1
  Mux3/1 -> Out4/1

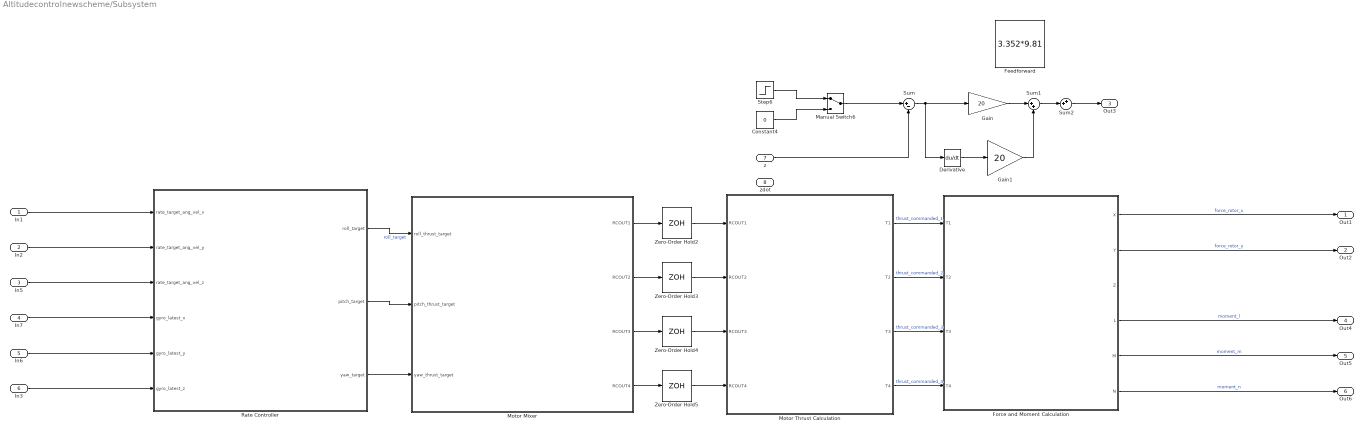
== system Altitudecontrolnewscheme/Subsystem ==
  In1 : Inport
  In2 : Inport  Port=2
  In5 : Inport  Port=3
  In7 : Inport  Port=4
  In6 : Inport  Port=5
  In3 : Inport  Port=6
  z : Inport  Port=7
  zdot : Inport  Port=8
  Constant4 : Constant  Value=0  SampleTime=0
  Derivative : Derivative
  "Feedforward " : Constant  Value=3.352*9.81
  Force and Moment Calculation : MATLAB Function  TreatAsAtomicUnit=on
  Gain : Gain  Gain=20
  Gain1 : Gain  Gain=20
  Manual Switch6 : ManualSwitch
  Motor Mixer : MATLAB Function  TreatAsAtomicUnit=on
  "Motor Thrust Calculation " : MATLAB Function  TreatAsAtomicUnit=on
  Rate Controller : MATLAB Function  TreatAsAtomicUnit=on
  Step6 : Step  Time=2  SampleTime=0
  Sum : Sum  Inputs=|+-
  Sum1 : Sum  Inputs=|++
  Sum2 : Sum  Inputs=++|
  Zero-Order Hold{2..5} (4 alike) : ZeroOrderHold  SampleTime=dtzoh
  Out1 : Outport
  Out2 : Outport  Port=2
  Out3 : Outport  Port=3
  Out4 : Outport  Port=4
  Out5 : Outport  Port=5
  Out6 : Outport  Port=6
  wires:
  Rate Controller/3(yaw_target) -> Motor Mixer/3(yaw_thrust_target)
  Rate Controller/1(roll_target) -> Motor Mixer/1(roll_thrust_target)  "roll_target"
  In5/1 -> Rate Controller/3(rate_target_ang_vel_z)
  In7/1 -> Rate Controller/4(gyro_latest_x)
  Force and Moment Calculation/2(Y) -> Out2/1  "force_rotor_y"
  Rate Controller/2(pitch_target) -> Motor Mixer/2(pitch_thrust_target)
  In2/1 -> Rate Controller/2(rate_target_ang_vel_y)
  In6/1 -> Rate Controller/5(gyro_latest_y)
  In3/1 -> Rate Controller/6(gyro_latest_z)
  In1/1 -> Rate Controller/1(rate_target_ang_vel_x)
  Force and Moment Calculation/4(L) -> Out4/1  "moment_l"
  Force and Moment Calculation/6(N) -> Out6/1  "moment_n"
  Force and Moment Calculation/5(M) -> Out5/1  "moment_m"
  Force and Moment Calculation/1(X) -> Out1/1  "force_rotor_x"
  Motor Mixer/4(RCOUT4) -> Zero-Order Hold5/1
  Motor Mixer/1(RCOUT1) -> Zero-Order Hold2/1
  Zero-Order Hold4/1 -> "Motor Thrust Calculation "/3(RCOUT3)
  Motor Mixer/2(RCOUT2) -> Zero-Order Hold3/1
  Zero-Order Hold3/1 -> "Motor Thrust Calculation "/2(RCOUT2)
  Zero-Order Hold5/1 -> "Motor Thrust Calculation "/4(RCOUT4)
  Motor Mixer/3(RCOUT3) -> Zero-Order Hold4/1
  Zero-Order Hold2/1 -> "Motor Thrust Calculation "/1(RCOUT1)
  "Motor Thrust Calculation "/1(T1) -> Force and Moment Calculation/1(T1)  "thrust_commanded_1"
  "Motor Thrust Calculation "/3(T3) -> Force and Moment Calculation/3(T3)  "thrust_commanded_3"
  "Motor Thrust Calculation "/2(T2) -> Force and Moment Calculation/2(T2)  "thrust_commanded_2"
  "Motor Thrust Calculation "/4(T4) -> Force and Moment Calculation/4(T4)  "thrust_commanded_4"
  Step6/1 -> Manual Switch6/1
  Constant4/1 -> Manual Switch6/2
  Manual Switch6/1 -> Sum/1
  z/1 -> Sum/2
  Derivative/1 -> Gain1/1
  Sum1/1 -> Sum2/2
  Gain/1 -> Sum1/1
  Sum/1 -> Gain/1, Derivative/1
  Gain1/1 -> Sum1/2
  Sum2/1 -> Out3/1

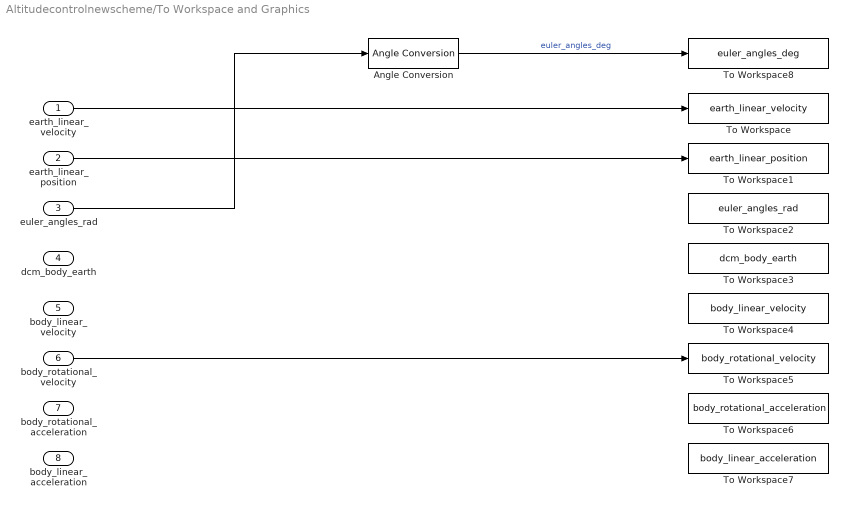
== system Altitudecontrolnewscheme/To Workspace and Graphics ==
  earth_linear_velocity : Inport
  earth_linear_position : Inport  Port=2
  euler_angles_rad : Inport  Port=3
  dcm_body_earth : Inport  Port=4
  body_linear_velocity : Inport  Port=5
  body_rotational_velocity : Inport  Port=6
  body_rotational_acceleration : Inport  Port=7
  body_linear_acceleration : Inport  Port=8
  Angle Conversion : aerolibconvert2/Angle Conversion  IU=rad  OU=deg
  To Workspace : ToWorkspace  VariableName=earth_linear_velocity  SampleTime=-1
  To Workspace1 : ToWorkspace  VariableName=earth_linear_position  SampleTime=-1
  To Workspace2 : ToWorkspace  VariableName=euler_angles_rad  SampleTime=-1
  To Workspace3 : ToWorkspace  VariableName=dcm_body_earth  SampleTime=-1
  To Workspace4 : ToWorkspace  VariableName=body_linear_velocity  SampleTime=-1
  To Workspace5 : ToWorkspace  VariableName=body_rotational_velocity  SampleTime=-1
  To Workspace6 : ToWorkspace  VariableName=body_rotational_acceleration  SampleTime=-1
  To Workspace7 : ToWorkspace  VariableName=body_linear_acceleration  SampleTime=-1
  To Workspace8 : ToWorkspace  VariableName=euler_angles_deg  SampleTime=-1
  wires:
  body_rotational_velocity/1 -> To Workspace5/1
  Angle Conversion/1 -> To Workspace8/1  "euler_angles_deg"
  euler_angles_rad/1 -> Angle Conversion/1
  earth_linear_position/1 -> To Workspace1/1
  earth_linear_velocity/1 -> To Workspace/1

== matlab function Altitudecontrolnewscheme/Subsystem/Rate Controller ==
  data: rate_target_ang_vel_x input; rate_target_ang_vel_y input; rate_target_ang_vel_z input; gyro_latest_x input; gyro_latest_y input; gyro_latest_z input; roll_target output; pitch_target output; yaw_target output; throttle_rpy_mix data_store_memory; throttle_rpy_mix_desired data_store_memory; dt data_store_memory; roll_rate_error_rads data_store_memory; roll_rate_last_input data_store_memory; roll_rate_filt_hz data_store_memory; roll_rate_derivative data_store_memory; roll_rate_integrator data_store_memory; roll_rate_kI data_store_memory; roll_rate_kP data_store_memory; roll_rate_kD data_store_memory; roll_rate_imax data_store_memory; roll_rate_proportional data_store_memory; limit_roll_pitch data_store_memory; pitch_rate_error_rads data_store_memory; pitch_rate_last_input data_store_memory; pitch_rate_filt_hz data_store_memory; pitch_rate_derivative data_store_memory; pitch_rate_integrator data_store_memory; pitch_rate_kI data_store_memory; pitch_rate_kP data_store_memory; pitch_rate_kD data_store_memory; pitch_rate_imax data_store_memory; pitch_rate_proportional data_store_memory; yaw_rate_error_rads data_store_memory; yaw_rate_last_input data_store_memory; yaw_rate_filt_hz data_store_memory; yaw_rate_derivative data_store_memory; yaw_rate_integrator data_store_memory; yaw_rate_kI data_store_memory; yaw_rate_kP data_store_memory; yaw_rate_kD data_store_memory; yaw_rate_imax data_store_memory; yaw_rate_proportional data_store_memory; limit_yaw data_store_memory
function [roll_target, pitch_target, yaw_target]  = rate_controller_run( rate_target_ang_vel_x, rate_target_ang_vel_y, rate_target_ang_vel_z , gyro_latest_x, gyro_latest_y, gyro_latest_z)
%RATE_CONTROLLER_RUN Summary of this function goes here
%   Detailed explanation goes here

update_throttle_rpy_mix();

roll_target = rate_target_to_motor_roll(gyro_latest_x, rate_target_ang_vel_x);
% roll_target = 0;
pitch_target = rate_target_to_motor_pitch(gyro_latest_y, rate_target_ang_vel_y);
% pitch_target = 0;
yaw_target = rate_target_to_motor_yaw(gyro_latest_z, rate_target_ang_vel_z);
% yaw_target = 0;
end

== matlab function Altitudecontrolnewscheme/Stabilise Attitude Controller ==
  data: pilot_throttle_in input; roll_rate_target output; pilot_roll_in input; pilot_pitch_in input; pilot_yaw_in input; pitch_rate_target output; yaw_rate_target output; roll_angle_latest input; ROLL_PITCH_INPUT_MAX data_store_memory; angle_max data_store_memory; throttle_avg_max data_store_memory; throttle_in data_store_memory; pitch_angle_latest input; acro_yaw_p data_store_memory; dt data_store_memory; rate_bf_ff_enabled data_store_memory; use_ff_and_input_shaping data_store_memory; attitude_target_quat data_store_memory; attitude_target_euler_angle_x data_store_memory; attitude_target_euler_angle_y data_store_memory; attitude_target_euler_angle_z data_store_memory; yaw_angle_latest input; gyro_latest_z input; attitude_target_euler_rate data_store_memory; AC_ATTITUDE_THRUST_ERROR_ANGLE data_store_memory; attitude_target_ang_vel data_store_memory; rate_target_ang_vel data_store_memory; thrust_error_angle data_store_memory; attitude_vehicle_quat data_store_memory; AC_ATTITUDE_ACCEL_Y_CONTROLLER_MAX_RADSS data_store_memory; yaw_attitude_kP data_store_memory; roll_attitude_kP data_store_memory; pitch_attitude_kP data_store_memory; throttle_rpy_mix data_store_memory
function [roll_rate_target, pitch_rate_target, yaw_rate_target]   = stabilise_run( pilot_throttle_in, pilot_roll_in, pilot_pitch_in, pilot_yaw_in, roll_angle_latest, pitch_angle_latest, yaw_angle_latest, gyro_latest_z)
%% stabilise_run
% 
% void Copter::stabilize_run()
% {
%     float target_roll, target_pitch;
%     float target_yaw_rate;
%     float pilot_throttle_scaled;
% 
%     // convert pilot input to lean angles
%     // To-Do: convert get_pilot_desired_lean_angles to return angles as floats
%     get_pilot_desired_lean_angles(channel_roll->get_control_in(), channel_pitch->get_control_in(), target_roll, target_pitch, aparm.angle_max);
% 
%     // get pilot's desired yaw rate
%     target_yaw_rate = get_pilot_desired_yaw_rate(channel_yaw->get_control_in());
% 
%     // get pilot's desired throttle
%     pilot_throttle_scaled = get_pilot_desired_throttle(channel_throttle->get_control_in());
% 
%     // call attitude controller
%     attitude_control.input_euler_angle_roll_pitch_euler_rate_yaw(target_roll, target_pitch, target_yaw_rate, get_smoothing_gain());
% 
%     // body-frame rate controller is run directly from 100hz loop
% 
%     // output pilot's throttle
%     attitude_control.set_throttle_out(pilot_throttle_scaled, true, g.throttle_filt);
% }
    %% Declare Global Variables
    global throttle_in throttle_avg_max
    
    %% Scale Pilot Inputs
    [roll_attitude_target_cd, pitch_attitude_target_cd] = get_pilot_desired_lean_angles(pilot_roll_in, pilot_pitch_in);
    yaw_rate_target = get_pilot_desired_yaw_rate(pilot_yaw_in);
    pilot_throttle_scaled = get_pilot_desired_throttle(pilot_throttle_in);
    
%     disp('roll_attitude_target');
%     disp(roll_attitude_target_cd);
%     disp(pitch_attitude_target);
%     disp(yaw_rate_target);
%     disp(pilot_throttle_in);
%      disp(pilot_throttle_scaled);
    %% Run the Attitude Controller

    [roll_rate_target, pitch_rate_target, yaw_rate_target] = input_euler_angle_roll_pitch_euler_rate_yaw(roll_attitude_target_cd, pitch_attitude_target_cd, yaw_rate_target, roll_angle_latest, pitch_angle_latest, yaw_angle_latest, gyro_latest_z);
    [throttle_in, throttle_avg_max] = set_throttle_out(pilot_throttle_scaled);
    
%     disp('roll_rate_target')
%     disp(roll_rate_target);
%     disp('roll_angle_latest')
%     disp(roll_angle_latest)
end

== matlab function Altitudecontrolnewscheme/Deltathrustloss ==
  data: ThrustPM input; dThrust output; time input
function dThrust  = dThrustLoss(ThrustPM,time)
%#Thrust to moments calculation

armLength = 0.41;                    %Meters
alpha = deg2rad(15);                 %Rad
chordLength = 0.040;                 %Meters
liftDragRatio = 0.1;

PercentageLoss1 = 50;
PercentageLoss2 = 0;
PercentageLoss3 = 0;
PercentageLoss4 = 0;

T1 = ThrustPM/100*PercentageLoss1;
T2 = ThrustPM/100*PercentageLoss2;
T3 = ThrustPM/100*PercentageLoss3;
T4 = ThrustPM/100*PercentageLoss4;

X = 0;
Y = 0;
Z = T1 + T2 + T3 + T4;

M = armLength * cos(alpha) * -((T2 + T4) - (T1 + T3));
L = armLength * sin(alpha) * ((T2 + T3) - (T1 + T4));
N = chordLength * ((T1 + T2) - (T3 + T4))/liftDragRatio;



dThrust = [0;
     0;
     0];

if time >= 4
    dThrust(1) = L;
    dThrust(2) = M;
    dThrust(3) = N;
end

%% Possibility to extend this disturbance dependent of distance to wall!

== matlab function Altitudecontrolnewscheme/Subsystem/Motor Mixer ==
  data: roll_thrust_target input; RCOUT1 output; pitch_thrust_target input; yaw_thrust_target input; RCOUT2 output; RCOUT3 output; RCOUT4 output; pwm_min data_store_memory; pwm_max data_store_memory; spin_min data_store_memory; spin_max data_store_memory; throttle_filter_cutoff_freq data_store_memory; throttle_filter_output data_store_memory; dt data_store_memory; yaw_allowed data_store_memory; throttle_thrust data_store_memory; throttle_avg_max data_store_memory; throttle_thrust_max data_store_memory; throttle_thrust_best_rpy data_store_memory; roll_factor data_store_memory; pitch_factor data_store_memory; yaw_factor data_store_memory; yaw_headroom data_store_memory; thrust_rpyt_out data_store_memory; throttle_in data_store_memory
function [RCOUT1, RCOUT2, RCOUT3, RCOUT4 ]  = motor_mixer( roll_thrust_target, pitch_thrust_target, yaw_thrust_target)
%% Motor Mixer

%
%   Matlab Implementation of the ArduPilot Motor Mixer
%   Outputs Motor Commands based on required rate targets
%
    global pwm_min pwm_max spin_min spin_max
    
    % Update throttle filter
    update_throttle_filter();

    % Update battery resistance
    % update_battery_resistance();
                                                                            %For the model, we will always assume we have maximum lift
    % Calc filtered battery voltage and lift_max
    % update_lift_max_from_batt_voltage();

    % Run spool logic
    % output_logic();
    
    % Calculate thrust
    thrust_rpyt_out = output_armed_stabilizing(roll_thrust_target, pitch_thrust_target, yaw_thrust_target);

    % Apply any thrust compensation for the frame
    % thrust_compensation();  %used for tilt rotors and tilt wings
    
    % Convert rpy_thrust values to pwm
%     RCOUT1 = pwm_min + (pwm_max-pwm_min)*(spin_min + (spin_max-spin_min)*thrust_rpyt_out(1));
%     RCOUT2 = pwm_min + (pwm_max-pwm_min)*(spin_min + (spin_max-spin_min)*thrust_rpyt_out(2));
%     RCOUT3 = pwm_min + (pwm_max-pwm_min)*(spin_min + (spin_max-spin_min)*thrust_rpyt_out(3));
%     RCOUT4 = pwm_min + (pwm_max-pwm_min)*(spin_min + (spin_max-spin_min)*thrust_rpyt_out(4));
    RCOUT1 = pwm_min + (pwm_max-pwm_min)*(spin_min + (spin_max-spin_min)*thrust_rpyt_out(1));
    RCOUT2 = pwm_min + (pwm_max-pwm_min)*(spin_min + (spin_max-spin_min)*thrust_rpyt_out(2));
    RCOUT3 = pwm_min + (pwm_max-pwm_min)*(spin_min + (spin_max-spin_min)*thrust_rpyt_out(3));
    RCOUT4 = pwm_min + (pwm_max-pwm_min)*(spin_min + (spin_max-spin_min)*thrust_rpyt_out(4));


    
% RCOUT1 = 1500;
% RCOUT2 = 1500;
% RCOUT3 = 1500;
% RCOUT4 = 1500;

 

end

== matlab function Altitudecontrolnewscheme/Subsystem/Force and Moment Calculation ==
  data: T1 input; X output; T2 input; T3 input; T4 input; Y output; Z output; L output; M output; N output
function [X, Y, Z, L, M, N] = forceMomentCalc(T1, T2, T3, T4)
%T1 = Motor 1 Thrust                (N)
%T2 = Motor 2 Thrust                (N)
%T3 = Motor 3 Thrust                (N)
%T4 = Motor 4 Thrust                (N)
%X = Force in x axis                (N)
%Y = Force in y axis                (N)                
%Z = Force in z axis                (N)
%L = Rolling moment around x axis   (N.m) Forward Positive
%M = Rolling moment around y axis   (N.m) Right Positive  
%N = Rolling moment around z axis   (N.m) CW Positive

%       ccw       cw            
%X         3    1
%           \  /
%            \/
%            /\
%           /  \
%          2    4       
%       cw        ccw   Y
%%%%%%%%%%%%%%%%%%%%%%%%%
armLength = 0.41;                    %Meters
alpha = deg2rad(15);                 %Rad
chordLength = 0.040;                 %Meters
liftDragRatio = 0.1;


X = 0;
Y = 0;
Z = T1 + T2 + T3 + T4;

M = armLength * cos(alpha) * -((T2 + T4) - (T1 + T3));
L = armLength * sin(alpha) * ((T2 + T3) - (T1 + T4));
N = chordLength * ((T1 + T2) - (T3 + T4))/liftDragRatio;

== matlab function Altitudecontrolnewscheme/Subsystem/Motor Thrust Calculation  ==
  data: RCOUT1 input; T1 output; RCOUT2 input; RCOUT3 input; RCOUT4 input; T2 output; T3 output; T4 output
function [T1, T2, T3, T4] = motorOutputs(RCOUT1, RCOUT2, RCOUT3, RCOUT4)
%   RCOUTx = PWM Value out of the Autopilot                (1000us-2000us)
%   Tx = Thrust value produced by the motor/rotor pair     (N)
%
%   1.Calculate Tmax by adding overhead onto hover throttle
%   2.Map RCOUT values between 0 and 1
%   3.Multiply unity RCOUT value by Tmax

% Tmax = 2*(2.2*9.8);                                         % Overhead * (Drone3 Mass * Gravity)/number of rotors
%Tmax = 7 * 9.8 / 4;                                          % (Max Lift from website * Gravity)/number of rotors

% RCOUT1 = math_scale_values(RCOUT1, 1000, 2000, 0, 1);
% RCOUT2 = math_scale_values(RCOUT2, 1000, 2000, 0, 1);
% RCOUT3 = math_scale_values(RCOUT3, 1000, 2000, 0, 1);
% RCOUT4 = math_scale_values(RCOUT4, 1000, 2000, 0, 1);




%% Thrustprofiles

% y=a+b*x+c*x^2
a1 = 1.393666128052866e-05; b1 = -0.011561304396739; c1 = -5.241059895477592;
a2 = 1.520135833168069e-05; b2 = -0.014819490529974; c2 = -3.069708487015390;
a3 = 1.487222188885199e-05; b3 = -0.014151314098819; c3 = -3.400064896380763;
a4 = 1.687390195532662e-05; b4 = -0.020091967333676; c4 = 1.104620195159495;

% Thrustprofile1 = RCOUT1^2*a1+RCOUT1*b1+c1;
% Thrustprofile2 = RCOUT2^2*a2+RCOUT2*b2+c2;
% Thrustprofile3 = RCOUT3^2*a3+RCOUT3*b3+c3;
% Thrustprofile4 = RCOUT4^2*a4+RCOUT4*b4+c4;

% T1 = Thrustprofile1;
% T2 = Thrustprofile2;
% % T3 = Thrustprofile3*0.95; %efficiencyloss
% % T4 = Thrustprofile4*0.95; %efficiencyloss
% T3 = Thrustprofile3; %efficiencyloss
% T4 = Thrustprofile4; %efficiencyloss


Thrustprofile1 = RCOUT1^2*a1+RCOUT1*b1+c1;
Thrustprofile2 = RCOUT2^2*a1+RCOUT2*b1+c1;
Thrustprofile3 = RCOUT3^2*a1+RCOUT3*b1+c1;
Thrustprofile4 = RCOUT4^2*a1+RCOUT4*b1+c1;
T1 = Thrustprofile1;
T2 = Thrustprofile2;
T3 = Thrustprofile3;
T4 = Thrustprofile4;
%% Other ways to calculate thrust
% T1 = Tmax*RCOUT1*(0.25-0.2388+0.25);
% T2 = Tmax*RCOUT2*(0.25-0.2477+0.25);
% T3 = Tmax*RCOUT3*(0.25-0.2658+0.25);
% T4 = Tmax*RCOUT4*(0.25-0.2476+0.25);

% T1 = Tmax*RCOUT1*(0.25-0.212+0.25);
% T2 = Tmax*RCOUT2*(0.25-0.2438+0.25);
% T3 = Tmax*RCOUT3*(0.25-0.29+0.25);
% T4 = Tmax*RCOUT4*(0.25-0.2420+0.25);

% efficiencyfactor=[0.95 0.95 1 1];
% ESCfactor = [1 1 1 1];
% motorfactor = [1 1 1 1];
% 
% T1 = Tmax*RCOUT1*efficiencyfactor(1)*ESCfactor(1)*motorfactor(1);
% T2 = Tmax*RCOUT2*efficiencyfactor(2)*ESCfactor(2)*motorfactor(2);
% T3 = Tmax*RCOUT3*efficiencyfactor(3)*ESCfactor(3)*motorfactor(3);
% T4 = Tmax*RCOUT4*efficiencyfactor(4)*ESCfactor(4)*motorfactor(4);

% T1 = Tmax*RCOUT1;
% T2 = Tmax*RCOUT2;
% T3 = Tmax*RCOUT3;
% T4 = Tmax*RCOUT4;
